simulink model "test_model"  (Simulink 8.4)
settings: Solver=ode45  StartTime=0.0  StopTime=10.0  RelTol=1e-3
settings Model: Creator=johnhung  LastModifiedBy=johnhung

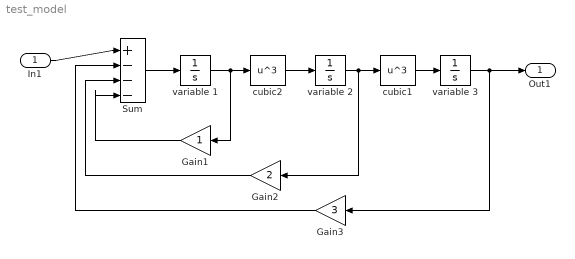
== system test_model ==
  In1 : Inport
  Gain1 : Gain
  Gain2 : Gain  Gain=2
  Gain3 : Gain  Gain=3
  Sum : Sum  Inputs=|+---
  cubic1 : Fcn  Expr=u^3
  cubic2 : Fcn  Expr=u^3
  variable 1 : Integrator
  variable 2 : Integrator
  variable 3 : Integrator
  Out1 : Outport
  wires:
  variable 1/1 -> cubic2/1, Gain1/1
  variable 2/1 -> cubic1/1, Gain2/1
  variable 3/1 -> Out1/1, Gain3/1
  Sum/1 -> variable 1/1
  In1/1 -> Sum/1
  Gain1/1 -> Sum/4
  Gain2/1 -> Sum/3
  Gain3/1 -> Sum/2
  cubic2/1 -> variable 2/1
  cubic1/1 -> variable 3/1
